simulink model "task_5_const"  (R2017a)
settings: Solver=FixedStepAuto  StartTime=0.0  StopTime=20  FixedStep=0.001  RelTol=1e-3
values from neighbouring files (symbols this model uses):
  K_d = 2*(2*zeta*omega) - 1    [task_3_const.m]    (also in task_3_dynamic.m; task_4_const.m; task_5.m)
  K_i = 50    [task_4_const.m]    (also in task_5.m = 500)
  K_p = 2*omega^2    [task_3_const.m]    (also in task_3_dynamic.m; task_4_const.m; task_5.m)
  r = 50    [constants.m]
  saturation = 20    [task_5.m]
  Tl = 500    [constants.m]
settings Model: Creator=evenmas  LastModifiedBy=evenmas

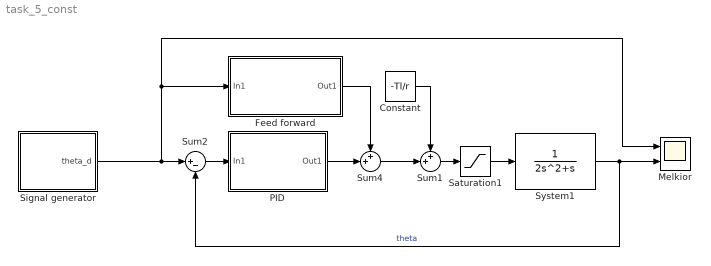
== system task_5_const ==
  Constant : Constant  Value=-Tl/r
  Feed forward : Subsystem
  "Melkior " : Scope  NumInputPorts=2
  PID : Subsystem
  Saturation1 : Saturate  UpperLimit=saturation  LowerLimit=-saturation  ZeroCross=off
  "Signal generator " : Subsystem
  Sum1 : Sum  Inputs=++|
  Sum2 : Sum  Inputs=|+-
  Sum4 : Sum  Inputs=++|
  System1 : TransferFcn  Denominator=[2 1 0]
  wires:
  System1/1 -> "Melkior "/2, Sum2/2  "theta"
  "Signal generator "/1(theta_d) -> "Melkior "/1, Feed forward/1(In1), Sum2/1
  Feed forward/1(Out1) -> Sum4/1
  Sum2/1 -> PID/1(In1)
  PID/1(Out1) -> Sum4/2
  Sum4/1 -> Sum1/2
  Sum1/1 -> Saturation1/1
  Constant/1 -> Sum1/1
  Saturation1/1 -> System1/1

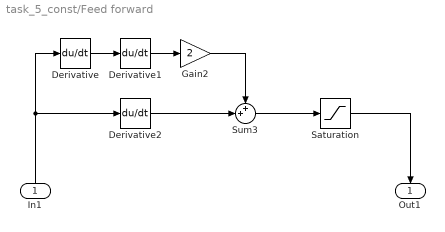
== system task_5_const/Feed forward ==
  In1 : Inport
  Derivative : Derivative
  Derivative1 : Derivative
  Derivative2 : Derivative
  Gain2 : Gain  Gain=2
  Saturation : Saturate  UpperLimit=20  LowerLimit=-20  ZeroCross=off
  Sum3 : Sum  Inputs=++|
  Out1 : Outport
  wires:
  Derivative2/1 -> Sum3/2
  Gain2/1 -> Sum3/1
  Derivative/1 -> Derivative1/1
  Derivative1/1 -> Gain2/1
  Sum3/1 -> Saturation/1
  In1/1 -> Derivative/1, Derivative2/1
  Saturation/1 -> Out1/1

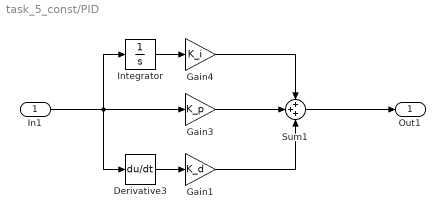
== system task_5_const/PID ==
  In1 : Inport
  Derivative3 : Derivative
  Gain1 : Gain  Gain=K_d
  Gain3 : Gain  Gain=K_p
  Gain4 : Gain  Gain=K_i
  Integrator : Integrator
  Sum1 : Sum  Inputs=+++
  Out1 : Outport
  wires:
  Gain3/1 -> Sum1/2
  Sum1/1 -> Out1/1
  Gain4/1 -> Sum1/1
  In1/1 -> Derivative3/1, Gain3/1, Integrator/1
  Derivative3/1 -> Gain1/1
  Gain1/1 -> Sum1/3
  Integrator/1 -> Gain4/1

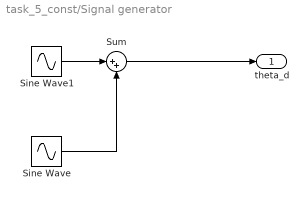
== system task_5_const/Signal generator  ==
  Sine Wave : Sin  Frequency=2  Phase=pi/2  SampleTime=0
  Sine Wave1 : Sin  SampleTime=0
  Sum : Sum  Inputs=|++
  theta_d : Outport
  wires:
  Sum/1 -> theta_d/1
  Sine Wave1/1 -> Sum/1
  Sine Wave/1 -> Sum/2
